simulink model "lab3_1"  (R2023a)
settings: Solver=VariableStepAuto  StartTime=0.0  StopTime=10  RelTol=1e-3
undefined symbols (not defined in the file or in its folder): C, K, L, u0, x0
settings Model: Creator=bz  LastModifiedBy=bz

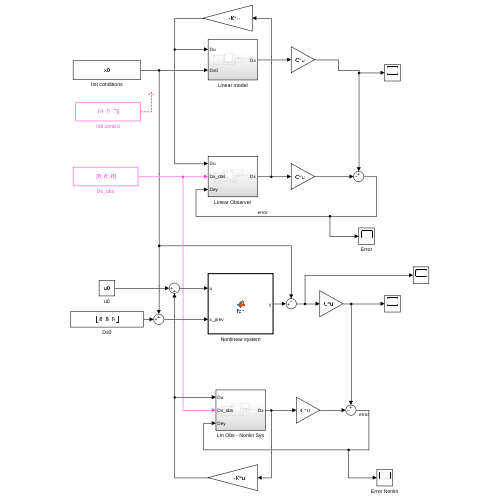
[thumbnail: Simulink's stored preview of the top-level diagram]
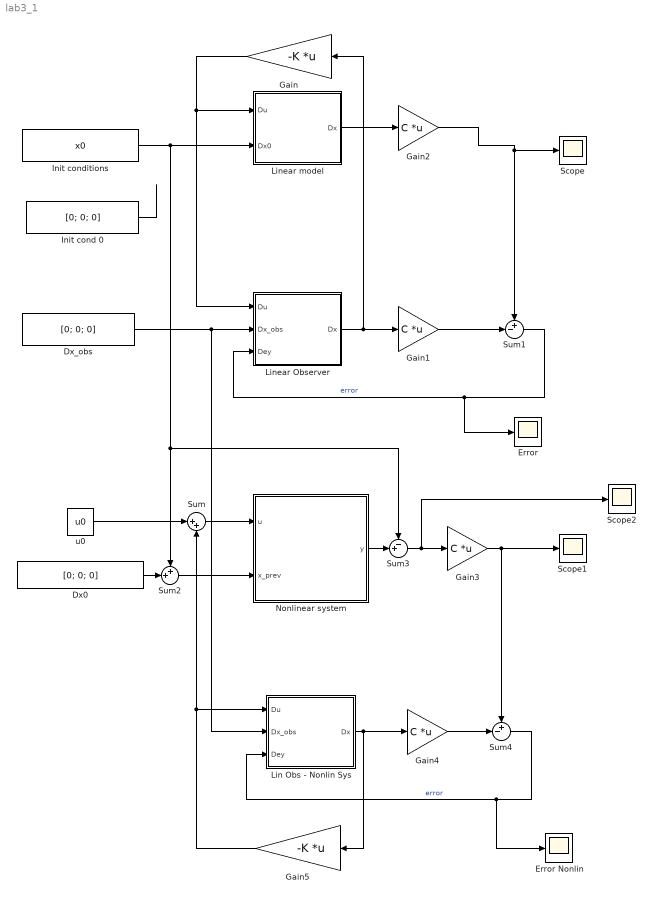
== system lab3_1 ==
  Dx0 : Constant  Value=[0; 0; 0]
  Dx_obs : Constant  Value=[0; 0; 0]  VectorParams1D=off
  Error : Scope
  Error Nonlin : Scope
  Gain : Gain  Gain=-K  Multiplication=Matrix(K*u)
  Gain{1..4} (4 alike) : Gain  Gain=C  Multiplication=Matrix(K*u)
  Gain5 : Gain  Gain=-K  Multiplication=Matrix(K*u)
  Init cond 0 : Constant  Value=[0; 0; 0]  VectorParams1D=off
  Init conditions : Constant  Value=x0  VectorParams1D=off
  Lin Obs - Nonlin Sys : Subsystem
  Linear Observer : Subsystem
  Linear model : Subsystem
  Nonlinear system : MATLAB Function  TreatAsAtomicUnit=on
  Scope : Scope
  Scope1 : Scope
  Scope2 : Scope
  Sum : Sum  Inputs=|++
  Sum1 : Sum  Inputs=+-|
  Sum2 : Sum  Inputs=++|
  Sum3 : Sum  Inputs=-+|
  Sum4 : Sum  Inputs=+-|
  u0 : Constant  Value=u0
  wires:
  Gain/1 -> Linear model/1(Du), Linear Observer/1(Du)
  Linear Observer/1(Dx) -> Gain/1, Gain1/1
  Init conditions/1 -> Linear model/2(Dx0), Sum3/1, Sum2/1
  Dx_obs/1 -> Lin Obs - Nonlin Sys/2(Dx_obs), Linear Observer/2(Dx_obs)
  Linear model/1(Dx) -> Gain2/1
  Gain1/1 -> Sum1/2
  Gain2/1 -> Scope/1, Sum1/1
  Sum1/1 -> Error/1, Linear Observer/3(Dey)  "error"
  Sum/1 -> Nonlinear system/1(u)
  Dx0/1 -> Sum2/2
  Sum2/1 -> Nonlinear system/2(x_prev)
  Nonlinear system/1(y) -> Sum3/2
  Sum3/1 -> Scope2/1, Gain3/1
  Lin Obs - Nonlin Sys/1(Dx) -> Gain5/1, Gain4/1
  Gain4/1 -> Sum4/2
  Gain3/1 -> Scope1/1, Sum4/1
  u0/1 -> Sum/1
  Gain5/1 -> Lin Obs - Nonlin Sys/1(Du), Sum/2
  Sum4/1 -> Error Nonlin/1, Lin Obs - Nonlin Sys/3(Dey)  "error"
  Init cond 0/1 -> ?

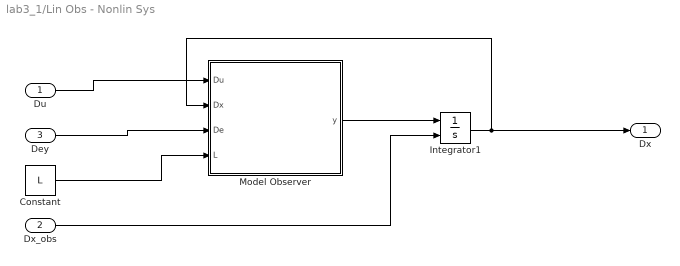
== system lab3_1/Lin Obs - Nonlin Sys ==
  Du : Inport
  Dx_obs : Inport  Port=2
  Dey : Inport  Port=3
  Constant : Constant  Value=L
  Integrator1 : Integrator  InitialConditionSource=external
  Model Observer : MATLAB Function  TreatAsAtomicUnit=on
  Dx : Outport
  wires:
  Model Observer/1(y) -> Integrator1/1
  Dx_obs/1 -> Integrator1/2
  Integrator1/1 -> Dx/1, Model Observer/2(Dx)
  Du/1 -> Model Observer/1(Du)
  Dey/1 -> Model Observer/3(De)
  Constant/1 -> Model Observer/4(L)

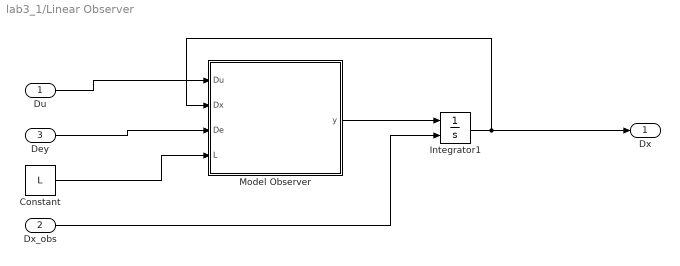
== system lab3_1/Linear Observer ==
  Du : Inport
  Dx_obs : Inport  Port=2
  Dey : Inport  Port=3
  Constant : Constant  Value=L
  Integrator1 : Integrator  InitialConditionSource=external
  Model Observer : MATLAB Function  TreatAsAtomicUnit=on
  Dx : Outport
  wires:
  Model Observer/1(y) -> Integrator1/1
  Dx_obs/1 -> Integrator1/2
  Integrator1/1 -> Dx/1, Model Observer/2(Dx)
  Du/1 -> Model Observer/1(Du)
  Dey/1 -> Model Observer/3(De)
  Constant/1 -> Model Observer/4(L)

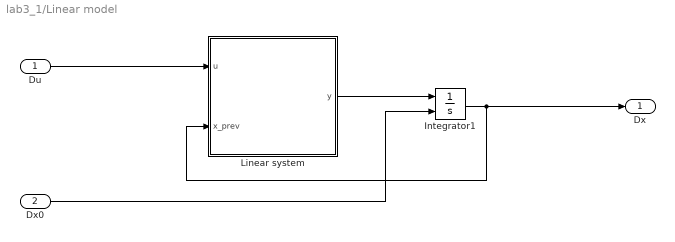
== system lab3_1/Linear model ==
  Du : Inport
  Dx0 : Inport  Port=2
  Integrator1 : Integrator  InitialConditionSource=external
  Linear system : MATLAB Function  TreatAsAtomicUnit=on
  Dx : Outport
  wires:
  Linear system/1(y) -> Integrator1/1
  Dx0/1 -> Integrator1/2
  Integrator1/1 -> Dx/1, Linear system/2(x_prev)
  Du/1 -> Linear system/1(u)

== matlab function lab3_1/Linear model/Linear system ==
  data: u input; y output size=[3,1]; x_prev input
function y  = fcn(u, x_prev)

A = [0              0.0010      0;
     1.6847         0           -0.0257;
     0              0           -0.2888] * 1e3;

B = [0;
     0;
     1.2706] * 1e3;

y = A * x_prev + B * u;

end

== matlab function lab3_1/Linear Observer/Model Observer ==
  data: Du input; y output size=[3,1]; Dx input; De input; L input
function y  = observer(Du, Dx, De, L)

A = [0              0.0010      0;
     1.6847         0           -0.0257;
     0              0           -0.2888] * 1e3;

B = [0;
     0;
     1.2706] * 1e3;

y = A * Dx + B * Du + L * De;

end

== matlab function lab3_1/Nonlinear system ==
  data: u input; y output size=[3,1]; x_prev input
function y  = fcn(u, x_prev)

% x_prev
x1 = x_prev(1);
% if x1 < 0
%     x1 = 0;
% end
x2 = x_prev(2);
x3 = x_prev(3);

FemP1 = 0.017521;
FemP2 = 0.0058231;

ci = -0.4;
ki = 4.4;
m = 0.016;
g = 9.81;

fiP1 = 1.4142e-4;
fiP2 = 4.5626e-3;

x1_dot = x2;
x2_dot = -(x3^2)*(FemP1/(FemP2*2*m))*exp(-x1/FemP2)+g;
x3_dot = 1/((fiP1/fiP2)*exp(-x1/fiP2))*(ki*u+ci-x3);

y = [x1_dot; x2_dot; x3_dot];

end

== matlab function lab3_1/Lin Obs - Nonlin Sys/Model Observer ==
  data: Du input; y output size=[3,1]; Dx input; De input; L input
function y  = observer(Du, Dx, De, L)

A = [0              0.0010      0;
     1.6847         0           -0.0257;
     0              0           -0.2888] * 1e3;

B = [0;
     0;
     1.2706] * 1e3;

y = A * Dx + B * Du + L * De;

end
